simulink model "im_foc_dcontrol_fixed_point"  (R2022b)
settings: Solver=FixedStepAuto  StartTime=0.0  StopTime=2  FixedStep=0.001  RelTol=1e-3
values from neighbouring files (symbols this model uses):
  B = 0.00825    [IM_System_1.m]    (also in IM_System_2.m; IM_System_3.m; IM_System_noPU_4p2p2kw.m; IM_System_noPU_4p2p2kw_1.m)
  J = 0.013    [IM_System_1.m]    (also in IM_System_2.m; IM_System_3.m; IM_System_noPU_4p2p2kw.m; IM_System_noPU_4p2p2kw_1.m)
  Lm = 0.245/3    (= 0.0816666666667)    [IM_System_1.m]    (also in IM_System_2.m; IM_System_3.m; IM_System_noPU_4p2p2kw.m; IM_System_noPU_4p2p2kw_1.m)
  Lr = Ls    (= 0.0852333333333)    [IM_System_1.m]    (also in IM_System_2.m; IM_System_3.m; IM_System_noPU_4p2p2kw.m; IM_System_noPU_4p2p2kw_1.m)
  Ls = 0.2557/3    (= 0.0852333333333)    [IM_System_1.m]    (also in IM_System_2.m; IM_System_3.m; IM_System_noPU_4p2p2kw.m; IM_System_noPU_4p2p2kw_1.m)
  pole = 4    [im_params.m]
  Rs = 2.5/3    (= 0.833333333333)    [IM_System_1.m]    (also in IM_System_2.m; IM_System_3.m; IM_System_noPU_4p2p2kw.m; IM_System_noPU_4p2p2kw_1.m)
  Tr = Lr/Rr    (= 0.139726775956)    [IM_System_1.m]    (also in IM_System_2.m; IM_System_3.m; IM_System_noPU_4p2p2kw.m; IM_System_noPU_4p2p2kw_1.m)
undefined symbols (not defined in the file or in its folder): sigbuilder_block, sigma
settings Model: Creator=jack  LastModifiedBy=jack

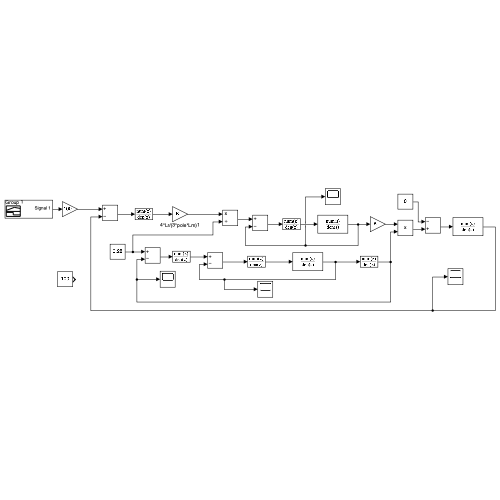
[thumbnail: Simulink's stored preview of the top-level diagram]
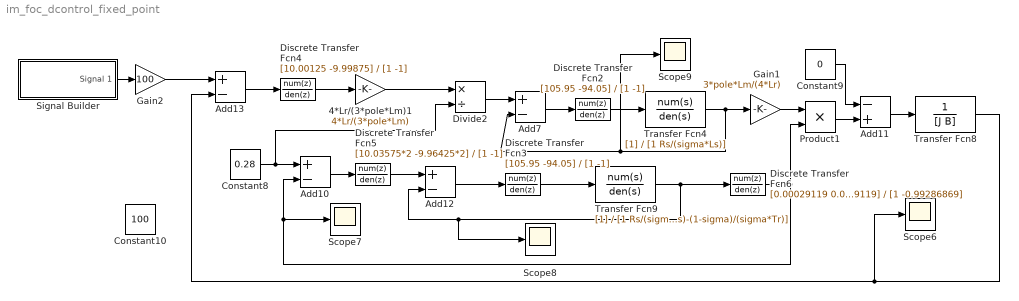
== system im_foc_dcontrol_fixed_point ==
  4*Lr/(3*pole*Lm)1 : Gain  Gain=4*Lr/(3*pole*Lm)
  Add{7,10,12..13} (4 alike) : Sum  Inputs=+-
  Add11 : Sum  Inputs=-+
  Constant10 : Constant  Value=100
  Constant8 : Constant  Value=0.28
  Constant9 : Constant  Value=0
  Discrete Transfer Fcn2 : DiscreteTransferFcn  Numerator=[105.95 -94.05]  Denominator=[1 -1]  SampleTime=0.001
  Discrete Transfer Fcn3 : DiscreteTransferFcn  Numerator=[105.95 -94.05]  Denominator=[1 -1]  SampleTime=0.001
  Discrete Transfer Fcn4 : DiscreteTransferFcn  Numerator=[10.00125 -9.99875]  Denominator=[1 -1]  SampleTime=0.001
  Discrete Transfer Fcn5 : DiscreteTransferFcn  Numerator=[10.03575*2 -9.96425*2]  Denominator=[1 -1]  SampleTime=0.001
  Discrete Transfer Fcn6 : DiscreteTransferFcn  Numerator=[0.00029119 0.00029119]  Denominator=[1 -0.99286869]  SampleTime=0.001
  Divide2 : Product  Inputs=*/
  Gain1 : Gain  Gain=3*pole*Lm/(4*Lr)
  Gain2 : Gain  Gain=100
  Product1 : Product
  Scope{6..9} (4 alike) : Scope
  Signal Builder : Subsystem  Tag=STV Subsys  LoadFcn=sigbuilder_block('load');  StartFcn=sigbuilder_block('start');  StopFcn=sigbuilder_block('stop');  ClipboardFcn=sigbuilder_block('clipboard');  mask(Sigbuilder block){tuvar=[0:10]}
      mask help: Simulink:masks:SigbuilderBlock_MD
      mask init:
      | if ~strcmp(get_param(bdroot(gcbh),'SimulationStatus'),'stopped') tuvar = sigbuilder_block('maskInit'); end
      settings: CopyFcn=sigbuilder_block('copy');  DeleteFcn=sigbuilder_block('delete');  ModelCloseFcn=sigbuilder_block('modelClose');  PreSaveFcn=sigbuilder_block('preSave');  PauseFcn=sigbuilder_block('pause');  ContinueFcn=sigbuilder_block('continue');  NameChangeFcn=sigbuilder_block('namechange');  OpenFcn=sigbuilder_block('open',[437.6 199.2 550.4 400 ]);  CloseFcn=sigbuilder_block('close');
      mask Display: plot(0, 0, 100, 100,[2, 2, 32, 32, 2], [68, 8, 8, 68, 68],[32, 2], [38, 38], [32, 19, 2],[53, 60, 44], [32, 17, 17, 2],[16, 16, 31, 31]);txt = getActiveGroup(gcbh);text(2, 100, txt,'verticalAlignment', 'top');
  Transfer Fcn4 : TransferFcn  Denominator=[1 Rs/(sigma*Ls)]
  Transfer Fcn8 : TransferFcn  Denominator=[J B]
  Transfer Fcn9 : TransferFcn  Denominator=[1 Rs/(sigma*Ls)-(1-sigma)/(sigma*Tr)]
  wires:
  Add7/1 -> Discrete Transfer Fcn2/1
  Divide2/1 -> Add7/1
  Add12/1 -> Discrete Transfer Fcn3/1
  Product1/1 -> Add11/2
  Add10/1 -> Discrete Transfer Fcn5/1
  Discrete Transfer Fcn3/1 -> Transfer Fcn9/1
  Discrete Transfer Fcn5/1 -> Add12/1
  Signal Builder/1(Signal 1) -> Gain2/1
  Discrete Transfer Fcn2/1 -> Transfer Fcn4/1
  Transfer Fcn4/1 -> Scope9/1, Add7/2, Gain1/1
  Gain1/1 -> Product1/1
  Discrete Transfer Fcn4/1 -> 4*Lr/(3*pole*Lm)1/1
  Transfer Fcn9/1 -> Discrete Transfer Fcn6/1, Scope8/1, Add12/2
  Add11/1 -> Transfer Fcn8/1
  4*Lr/(3*pole*Lm)1/1 -> Divide2/1
  Constant8/1 -> Add10/1, Divide2/2
  Constant9/1 -> Add11/1
  Transfer Fcn8/1 -> Scope6/1, Add13/2
  Discrete Transfer Fcn6/1 -> Scope7/1, Add10/2, Product1/2
  Add13/1 -> Discrete Transfer Fcn4/1
  Gain2/1 -> Add13/1

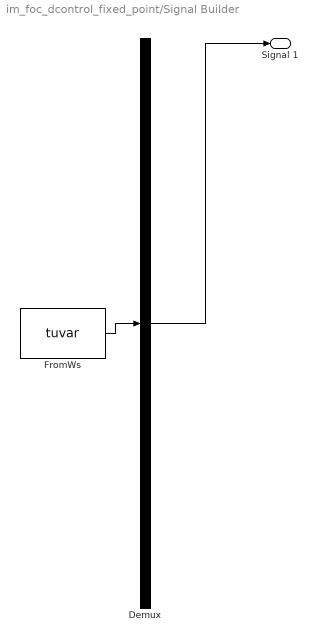
== system im_foc_dcontrol_fixed_point/Signal Builder ==
  Demux : Demux  Tag=STV Demux  Outputs=1
      settings: DisplayOption=none
  FromWs : FromWorkspace  Tag=STV FromWs  VariableName=tuvar
      SigBuilderData=|
      | common.afterFinalStr = 'Extrapolate'
      | common.sampleTime = 0
      | dataSet.timeRange = [0 10]
      | dataSet.name = 'Group 1'
      | sbobj.Groups.Name = 'Group 1'
      | sbobj.Groups.Signals.Name = 'Signal 1'
      | sbobj.Groups.Signals.XData = [0 0.5 4 6 6 10]
      | sbobj.Groups.Signals.YData = [0 1 1 1 0 0]
  Signal 1 : Outport  Tag=STV Outport
  wires:
  Demux/1 -> Signal 1/1
  FromWs/1 -> Demux/1
